simulink model "es2_sim"  (R2023b)
settings: Solver=VariableStepAuto  StartTime=0.0  StopTime=5  RelTol=1e-3
values from neighbouring files (symbols this model uses):
  x0 = [3 5]'    [es2.m]    (also in es2_2.m = [3;5])
settings Model: Creator=stefa  LastModifiedBy=stefa

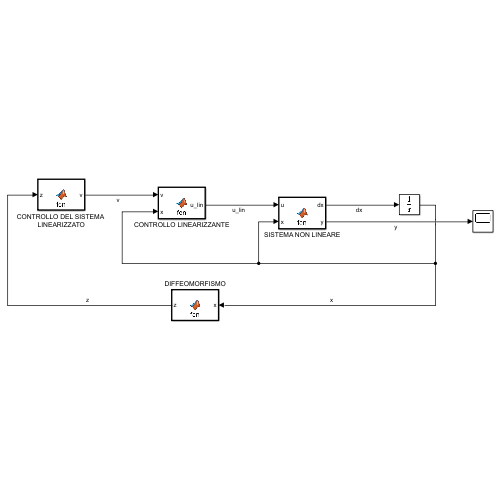
[thumbnail: Simulink's stored preview of the top-level diagram]
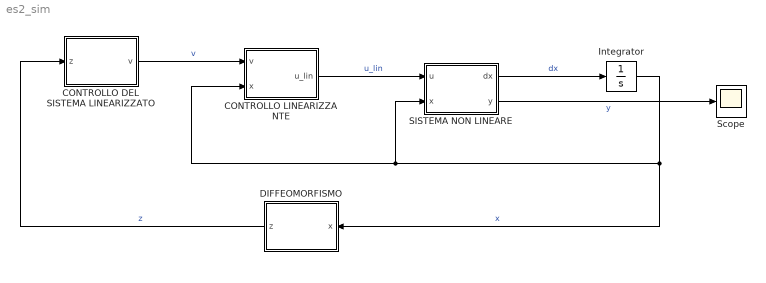
== system es2_sim ==
  CONTROLLO DEL SISTEMA LINEARIZZATO : MATLAB Function  TreatAsAtomicUnit=on
  CONTROLLO LINEARIZZANTE : MATLAB Function  TreatAsAtomicUnit=on
  DIFFEOMORFISMO : MATLAB Function  TreatAsAtomicUnit=on
  Integrator : Integrator  InitialCondition=x0
  SISTEMA NON LINEARE : MATLAB Function  TreatAsAtomicUnit=on
  Scope : Scope
  wires:
  Integrator/1 -> DIFFEOMORFISMO/1(x), SISTEMA NON LINEARE/2(x), CONTROLLO LINEARIZZANTE/2(x)  "x"
  CONTROLLO DEL SISTEMA LINEARIZZATO/1(v) -> CONTROLLO LINEARIZZANTE/1(v)  "v"
  DIFFEOMORFISMO/1(z) -> CONTROLLO DEL SISTEMA LINEARIZZATO/1(z)  "z"
  SISTEMA NON LINEARE/1(dx) -> Integrator/1  "dx"
  SISTEMA NON LINEARE/2(y) -> Scope/1  "y"
  CONTROLLO LINEARIZZANTE/1(u_lin) -> SISTEMA NON LINEARE/1(u)  "u_lin"

== matlab function es2_sim/SISTEMA NON LINEARE ==
  data: dx output; u input; y output; x input
function [dx,y]= fcn(u,x)
x1=x(1);
x2=x(2);
dx=[(x1^2+x1)*x2;-2*x2+x1-x2*u+6*u];
y = 5*x1;

== matlab function es2_sim/CONTROLLO DEL SISTEMA LINEARIZZATO ==
  data: z input; v output
function v = fcn(z)
K=[50 15];
v=-K*z;

== matlab function es2_sim/DIFFEOMORFISMO ==
  data: x input; z output
function z = fcn(x)
x1=x(1);
x2=x(2);
z =[5*x1;5*x2*(x1^2 + x1)];

== matlab function es2_sim/CONTROLLO LINEARIZZANTE ==
  data: v input; u_lin output; x input
function u_lin = fcn(v,x)

x1=x(1);
x2=x(2);

u_lin=((5*x1^2 + 5*x1)*(x1 - 2*x2) - v + 5*x2^2*(2*x1 + 1)*(x1^2 + x1))/((5*x1^2 + 5*x1)*(x2 - 6));
